simulink model "Test01"  (Simulink 5.0)
settings: Solver=ode45  StartTime=0.0  StopTime=inf  FixedStep=1/100000  MaxStep=1/100000  RelTol=1e-3
libraries: commcontsrc2 x2
settings Model: LastModifiedBy=Administrator  RTWOptions="-aEnforceIntegerDowncast=1 -aExtMode=0 -aExtModeTesting=0 -aFoldNonRolledExpr=1 -aForceParamTrailComments=0 -aGenerateComments=1 -aGenerateReport=0 -aIgnoreCustomStorageClasses=1 -aIncDataTypeInIds=0 -aIncHierarchyInIds=0 -aInlineInvariantSignals=1 -aInlineParameters=0 -aInlinedPrmAccess=\"Literals\" -aLocalBlockOutputs=1 -aLogVarNameModifier=\"rt_\" -aMaxRTWIdLen=31 -aPrefixModelToSubsysFcnNames=1 -aRTWVerbose=1 -aRollThreshold=5 -aShowEliminatedStatements=0"

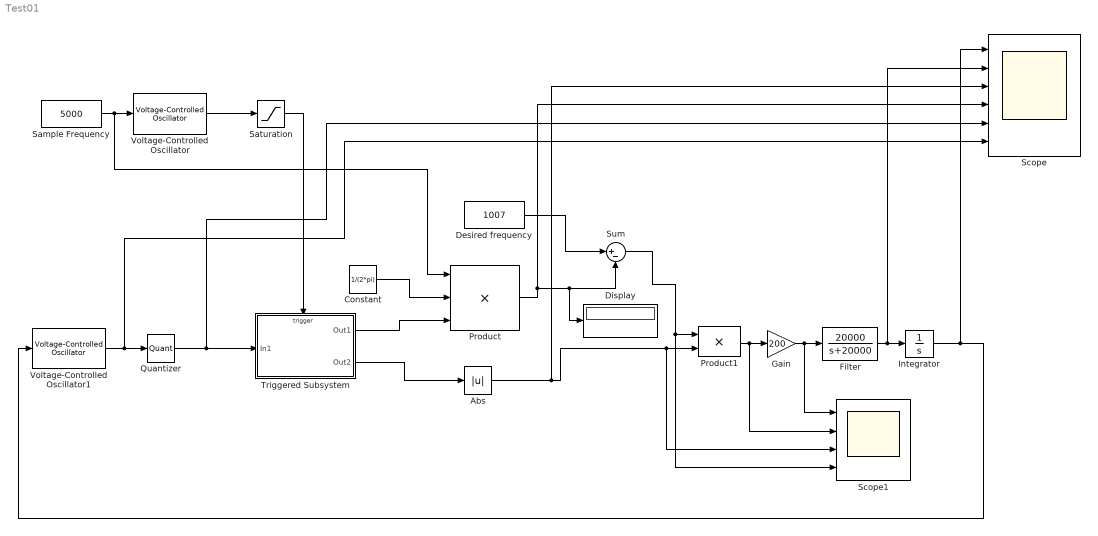
== system Test01 ==
  Abs : Abs  SaturateOnIntegerOverflow=on
  Constant : Constant  Value=1/(2*pi)
  Desired frequency : Constant  Value=1007
  Display : Display
  Filter : TransferFcn  Numerator=[20000]  Denominator=[1 20000]
  Gain : Gain  Gain=200  SaturateOnIntegerOverflow=on
  Integrator : Integrator
  Product : Product  Inputs=3  SaturateOnIntegerOverflow=on
  Product1 : Product  SaturateOnIntegerOverflow=on
  Quantizer : Quantizer  QuantizationInterval=2/(2^10)
  Sample Frequency : Constant  Value=5000
  Saturation : Saturate  UpperLimit=1  LowerLimit=-1
  Scope : Scope  NumInputPorts=6
      settings: TickLabels=on  TimeRange=0.003972194637537239  YMin=1006.93~-150~5.55112e-017~990~-1~-1  YMax=1006.98~125~1~1035~1~1
  Scope1 : Scope  NumInputPorts=4
      settings: TickLabels=on  TimeRange=0.00297914597815293  YMin=-175~-0.8~0.05~-5  YMax=125~0.7~1~2
  Sum : Sum  Inputs=|+-  SaturateOnIntegerOverflow=on
  Triggered Subsystem : Subsystem  TreatAsAtomicUnit=on
  Voltage-Controlled Oscillator : commcontsrc2/Voltage-Controlled Oscillator  Ac=100  Fc=0  Kc=1  Ph=0
  Voltage-Controlled Oscillator1 : commcontsrc2/Voltage-Controlled Oscillator  Ac=1  Fc=0  Kc=1  Ph=0
  wires:
  Voltage-Controlled Oscillator1/1 -> Quantizer/1, Scope/6
  Quantizer/1 -> Triggered Subsystem/1(In1), Scope/5
  Voltage-Controlled Oscillator/1 -> Saturation/1
  Triggered Subsystem/2(Out2) -> Abs/1
  Gain/1 -> Filter/1, Scope1/1
  Product1/1 -> Gain/1, Scope1/2
  Filter/1 -> Integrator/1, Scope/2
  Sample Frequency/1 -> Voltage-Controlled Oscillator/1, Product/1
  Saturation/1 -> Triggered Subsystem/Trigger
  Triggered Subsystem/1(Out1) -> Product/3
  Constant/1 -> Product/2
  Abs/1 -> Scope/3, Product1/2, Scope1/3
  Desired frequency/1 -> Sum/1
  Product/1 -> Scope/4, Sum/2, Display/1
  Sum/1 -> Product1/1, Scope1/4
  Integrator/1 -> Scope/1, Voltage-Controlled Oscillator1/1

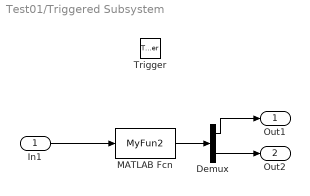
== system Test01/Triggered Subsystem ==
  In1 : Inport
  Trigger : TriggerPort
  Demux : Demux  Outputs=2
  MATLAB Fcn : MATLABFcn  MATLABFcn=MyFun2
  Out1 : Outport
  Out2 : Outport  Port=2
  wires:
  In1/1 -> MATLAB Fcn/1
  MATLAB Fcn/1 -> Demux/1
  Demux/1 -> Out1/1
  Demux/2 -> Out2/1
